simulink model "inverter_fault_rem_sim"  (R2016a)
settings: Solver=ode4  StartTime=0.0  StopTime=Tfinal  FixedStep=Ts  RelTol=1e-3
values from neighbouring files (symbols this model uses):
  Cdc = 200e-6    (= 0.0002)    [inverter_fault_sim.m]
  delta = acos(Ef/Vt)    [inverter_fault_sim.m]
  Ef = 160    [inverter_fault_sim.m]
  Foct = 0    [inverter_fault_sim.m]
  Focw = 1    [inverter_fault_sim.m]
  fout = Nr*p/60    (= 100)    [inverter_fault_sim.m]
  Fsct = 0    [inverter_fault_sim.m]
  Fscw = 0    [inverter_fault_sim.m]
  Ls = 3e-3    (= 0.003)    [inverter_fault_sim.m]    (also in short_circuit.m = 0.00365)
  ma = Vt*sqrt(3)/(Vdcm*0.612)    [inverter_fault_sim.m]
  phase = 0*pi/180    (= 0)    [fault_tolerance_torque.m]    (also in inverter_fault_sim.m = [0 90 0 90])
  Rin = 10    [inverter_fault_sim.m]
  Ripth = 0.15    [inverter_fault_sim.m]
  Rs = 0.277e-6    (= 2.77e-07)    [inverter_fault_sim.m]    (also in short_circuit.m = 0.277)
  Tfault = 0    [inverter_fault_sim.m]
  Ts = 1e-6    (= 1e-06)    [inverter_fault_sim.m]
  Vin = Vdc + Rin*(Pout/Vdc)    (= 688.148148148)    [inverter_fault_sim.m]
  wm = Nm*2*pi/60    (= 62.8318530718)    [fault_tolerance_torque.m]    (also in inverter_fault_sim.m)
  wout = 2*pi*fout    (= 628.318530718)    [inverter_fault_sim.m]
undefined symbols (not defined in the file or in its folder): Lload, Rload
libraries: powerlib x35, powerlib_meascontrol x7, simulink x2
settings Model: Creator=ugurm  LastModifiedBy=mesutto
settings DataIOCC: LimitDataPoints=on  SaveFormat=Array
settings DebuggingCC: UnderspecifiedInitializationDetection=Classic  MergeDetectMultiDrivingBlocksExec=none  SolverPrmCheckMsg=warning  StateNameClashWarn=warning
settings HardwareCC: ProdBitPerPointer=32  ProdLargestAtomicFloat=None  ProdIntDivRoundTo=Undefined  ProdEndianess=Unspecified  ProdWordSize=32  ProdHWDeviceType=32-bit Generic
settings ModelReferenceCC: PropagateSignalLabelsOutOfModel=off
settings ConfigComp: CovModelRefEnable=Off

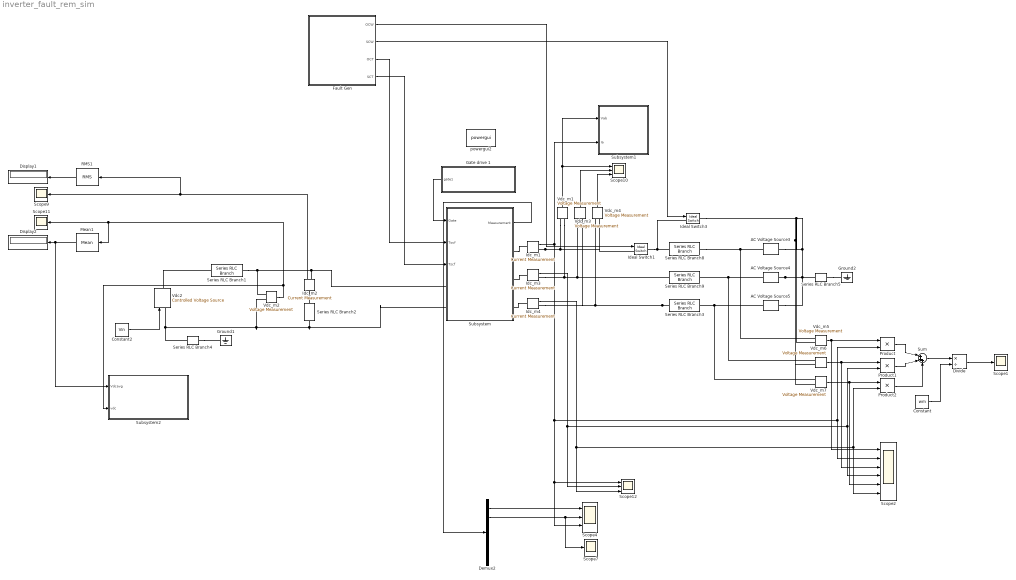
== system inverter_fault_rem_sim ==
  AC Voltage Source3 : powerlib/Electrical Sources/AC Voltage Source  Amplitude=Ef*sqrt(2)  Phase=0  Frequency=fout  SampleTime=0  Measurements=None  BusType=swing  Pref=10e3  Qref=0  Qmin=-inf  Qmax=+inf
  AC Voltage Source4 : powerlib/Electrical Sources/AC Voltage Source  Amplitude=Ef*sqrt(2)  Phase=-120  Frequency=fout  SampleTime=0  Measurements=None  BusType=swing  Pref=10e3  Qref=0  Qmin=-inf  Qmax=+inf
  AC Voltage Source5 : powerlib/Electrical Sources/AC Voltage Source  Amplitude=Ef*sqrt(2)  Phase=-240  Frequency=fout  SampleTime=0  Measurements=None  BusType=swing  Pref=10e3  Qref=0  Qmin=-inf  Qmax=+inf
  Constant : Constant  Value=wm
  Constant2 : Constant  Value=Vin
  Demux2 : Demux  Outputs=12
  Display1 : Display
  Display2 : Display
  Divide : Product  Inputs=*/
  Fault Gen : Subsystem
  Gate drive 1 : Subsystem
  Ground1 : powerlib/Elements/Ground  LConnTagsString=a
  Ground2 : powerlib/Elements/Ground  LConnTagsString=a
  Idc_m{1..4} (4 alike) : powerlib/Measurements/Current Measurement  PhasorSimulation=off  OutputType=Complex  PSBequivalent=0
  Ideal Switch1 : powerlib/Power Electronics/Ideal Switch  Ron=0.001  Lon=0  IC=0  Rs=1e9  Cs=inf  Measurements=off
  Ideal Switch3 : powerlib/Power Electronics/Ideal Switch  Ron=0.001  Lon=0  IC=0  Rs=1e9  Cs=inf  Measurements=off
  Mean1 : powerlib_meascontrol/Measurements/Mean  Freq=fout  Vinit=0  Ts=0
  Product : Product
  Product1 : Product
  Product2 : Product
  RMS1 : powerlib_meascontrol/Measurements/RMS  TrueRMS=on  Freq=fout  RMSInit=0  Ts=0
  Scope{1,7,9,11} (4 alike) : Scope
  Scope10 : Scope  NumInputPorts=3
  Scope12 : Scope  NumInputPorts=3
  Scope2 : Scope  NumInputPorts=6
  Scope4 : Scope  NumInputPorts=3
  Series RLC Branch1 : powerlib/Elements/Series RLC Branch  LConnTagsString=__new0  RConnTagsString=__new0  BranchType=R  Resistance=Rin  Inductance=Lload  SetiL0=off  InitialCurrent=0  Capacitance=1e-6  Setx0=off  InitialVoltage=0  Measurements=None
  Series RLC Branch2 : powerlib/Elements/Series RLC Branch  LConnTagsString=__new0  RConnTagsString=__new0  BranchType=C  Resistance=Rload  Inductance=Lload  SetiL0=off  InitialCurrent=0  Capacitance=Cdc  Setx0=off  InitialVoltage=0  Measurements=None
  Series RLC Branch3 : powerlib/Elements/Series RLC Branch  LConnTagsString=__new0  RConnTagsString=__new0  BranchType=RL  Resistance=Rs  Inductance=Ls  SetiL0=off  InitialCurrent=0  Capacitance=1e-6  Setx0=off  InitialVoltage=0  Measurements=None
  Series RLC Branch4 : powerlib/Elements/Series RLC Branch  LConnTagsString=__new0  RConnTagsString=__new0  BranchType=R  Resistance=1e12  Inductance=Lload  SetiL0=off  InitialCurrent=0  Capacitance=1e-6  Setx0=off  InitialVoltage=0  Measurements=None
  Series RLC Branch5 : powerlib/Elements/Series RLC Branch  LConnTagsString=__new0  RConnTagsString=__new0  BranchType=R  Resistance=1e12  Inductance=Lload  SetiL0=off  InitialCurrent=0  Capacitance=1e-6  Setx0=off  InitialVoltage=0  Measurements=None
  Series RLC Branch8 : powerlib/Elements/Series RLC Branch  LConnTagsString=__new0  RConnTagsString=__new0  BranchType=RL  Resistance=Rs  Inductance=Ls  SetiL0=off  InitialCurrent=0  Capacitance=1e-6  Setx0=off  InitialVoltage=0  Measurements=None
  Series RLC Branch9 : powerlib/Elements/Series RLC Branch  LConnTagsString=__new0  RConnTagsString=__new0  BranchType=RL  Resistance=Rs  Inductance=Ls  SetiL0=off  InitialCurrent=0  Capacitance=1e-6  Setx0=off  InitialVoltage=0  Measurements=None
  Subsystem : Subsystem
  Subsystem1 : Subsystem
  Subsystem2 : Subsystem
  Sum : Sum  Inputs=|+++
  Vdc2 : powerlib/Electrical Sources/Controlled Voltage Source  Initialize=off  Source_Type=DC  Amplitude=200  Phase=0  Frequency=0  Measurements=None
  Vdc_m{1..7} (7 alike) : powerlib/Measurements/Voltage Measurement  PhasorSimulation=off  OutputType=Complex  PSBequivalent=0
  powergui2 : powerlib/powergui  Priority=1  SimulationMode=Discrete  SolverType=Tustin  SampleTime=Ts  frequency=60  SPID=off  DisableSnubberDevices=off  DisableRonSwitches=off  DisableVfSwitches=off  SwTol=0  DisplayEquations=off  Interpol=off  ExternalGateDelay=off  methode=off  Ts=0  FunctionMessages=off  echomessages=off  HookPort=off  EnableUseOfTLC=off  x0status=blocks  frequencyindice=0  Pbase=100e6  ErrMax=1e-4  Iterations=50  UnitsV=kV  UnitsW=MW  buscounter=0  RestoreLinks=warning  ResistiveCurrentMeasurement=off  Frange=[0:2:500]  Ylog=off  Xlog=on  ShowGrid=off  save=off  variable=ZData  structure=Vdc  ZoomFFT=off  StartTime=0.04  cycles=5  DisplayStyle=5  fundamental=50  FreqAxis=off  MaxFrequency=30000  frequencyindicesteady=1  RmsSteady=1  display=off
  wires:
  Gate drive 1/1(gate1) -> Subsystem/1(Gate)
  Vdc_m1/1 -> Subsystem1/1(Vab), Scope10/1
  Idc_m1/1 -> Subsystem1/2(Ia), Product/2, Scope2/2, Scope4/3, Scope12/1
  Constant2/1 -> Vdc2/1
  Idc_m2/1 -> RMS1/1, Scope9/1
  Vdc_m2/1 -> Subsystem2/2(vdc), Mean1/1, Scope11/1
  Idc_m3/1 -> Scope12/2, Product1/2, Scope2/4
  Idc_m4/1 -> Product2/2, Scope2/6, Scope12/3
  RMS1/1 -> Display1/1
  Vdc_m3/1 -> Scope10/2
  Vdc_m4/1 -> Scope10/3
  Mean1/1 -> Subsystem2/1(Vdcavg), Display2/1
  Demux2/1 -> Scope4/1
  Demux2/3 -> Scope7/1, Scope4/2
  Subsystem/1(Measurement) -> Demux2/1
  Fault Gen/4(SCT) -> Subsystem/3(Tscf)
  Fault Gen/3(OCT) -> Subsystem/2(Tocf)
  Fault Gen/2(SCW) -> Ideal Switch3/1
  Fault Gen/1(OCW) -> Ideal Switch1/1
  Vdc_m5/1 -> Scope2/1, Product/1
  Vdc_m6/1 -> Scope2/3, Product1/1
  Vdc_m7/1 -> Scope2/5, Product2/1
  Product1/1 -> Sum/2
  Product2/1 -> Sum/3
  Product/1 -> Sum/1
  Sum/1 -> Divide/1
  Constant/1 -> Divide/2
  Divide/1 -> Scope1/1
  connections:
  Idc_m1/RConn1 -- Ideal Switch1/LConn1 -- Vdc_m4/LConn2 -- Vdc_m1/LConn1
  Series RLC Branch2/RConn1 -- Subsystem/LConn2 -- Vdc_m2/LConn2 -- Series RLC Branch4/LConn1 -- Vdc2/LConn1
  Series RLC Branch1/RConn1 -- Vdc_m2/LConn1 -- Subsystem/LConn1 -- Idc_m2/RConn1
  AC Voltage Source4/LConn1 -- Ideal Switch3/RConn1 -- Vdc_m7/LConn2 -- Vdc_m6/LConn2 -- Vdc_m5/LConn2 -- AC Voltage Source3/LConn1 -- Series RLC Branch5/LConn1 -- AC Voltage Source5/LConn1
  Series RLC Branch3/LConn1 -- Vdc_m4/LConn1 -- Idc_m4/RConn1 -- Vdc_m3/LConn2
  Vdc_m1/LConn2 -- Idc_m3/RConn1 -- Vdc_m3/LConn1 -- Series RLC Branch9/LConn1
  Subsystem/RConn1 -- Idc_m1/LConn1
  Idc_m4/LConn1 -- Subsystem/RConn3
  Series RLC Branch4/RConn1 -- Ground1/LConn1
  AC Voltage Source4/RConn1 -- Vdc_m6/LConn1 -- Series RLC Branch9/RConn1
  Idc_m3/LConn1 -- Subsystem/RConn2
  Idc_m2/LConn1 -- Series RLC Branch2/LConn1
  Vdc2/RConn1 -- Series RLC Branch1/LConn1
  AC Voltage Source5/RConn1 -- Vdc_m7/LConn1 -- Series RLC Branch3/RConn1
  Series RLC Branch5/RConn1 -- Ground2/LConn1
  Series RLC Branch8/RConn1 -- Vdc_m5/LConn1 -- AC Voltage Source3/RConn1
  Ideal Switch1/RConn1 -- Ideal Switch3/LConn1 -- Series RLC Branch8/LConn1

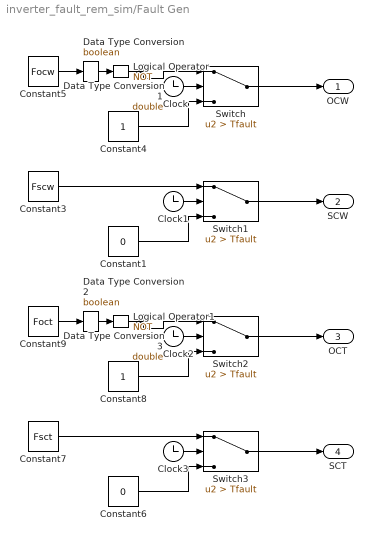
== system inverter_fault_rem_sim/Fault Gen ==
  Clock{,1..3} (4 alike) : Clock
  Constant1 : Constant  Value=0
  Constant3 : Constant  Value=Fscw
  Constant4 : Constant
  Constant5 : Constant  Value=Focw
  Constant6 : Constant  Value=0
  Constant7 : Constant  Value=Fsct
  Constant8 : Constant
  Constant9 : Constant  Value=Foct
  Data Type Conversion : DataTypeConversion  OutDataTypeStr=boolean
  Data Type Conversion1 : DataTypeConversion  OutDataTypeStr=double
  Data Type Conversion2 : DataTypeConversion  OutDataTypeStr=boolean
  Data Type Conversion3 : DataTypeConversion  OutDataTypeStr=double
  Logical Operator : Logic  Operator=NOT  AllPortsSameDT=off  OutDataTypeStr=boolean
  Logical Operator1 : Logic  Operator=NOT  AllPortsSameDT=off  OutDataTypeStr=boolean
  Switch{,1..3} (4 alike) : Switch  Criteria=u2 > Threshold  Threshold=Tfault
  OCW : Outport
  SCW : Outport  Port=2
  OCT : Outport  Port=3
  SCT : Outport  Port=4
  wires:
  Data Type Conversion1/1 -> Switch/1
  Data Type Conversion/1 -> Logical Operator/1
  Logical Operator/1 -> Data Type Conversion1/1
  Constant5/1 -> Data Type Conversion/1
  Constant1/1 -> Switch1/3
  Constant3/1 -> Switch1/1
  Clock1/1 -> Switch1/2
  Switch1/1 -> SCW/1
  Switch/1 -> OCW/1
  Constant4/1 -> Switch/3
  Clock/1 -> Switch/2
  Clock2/1 -> Switch2/2
  Clock3/1 -> Switch3/2
  Constant6/1 -> Switch3/3
  Switch2/1 -> OCT/1
  Data Type Conversion3/1 -> Switch2/1
  Constant9/1 -> Data Type Conversion2/1
  Constant8/1 -> Switch2/3
  Logical Operator1/1 -> Data Type Conversion3/1
  Data Type Conversion2/1 -> Logical Operator1/1
  Constant7/1 -> Switch3/1
  Switch3/1 -> SCT/1

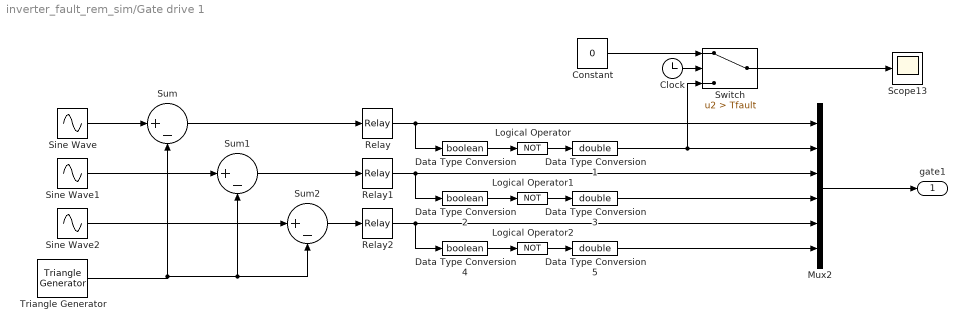
== system inverter_fault_rem_sim/Gate drive 1 ==
  Clock : Clock
  Constant : Constant  Value=0
  Data Type Conversion : DataTypeConversion  OutDataTypeStr=boolean
  Data Type Conversion1 : DataTypeConversion  OutDataTypeStr=double
  Data Type Conversion2 : DataTypeConversion  OutDataTypeStr=boolean
  Data Type Conversion3 : DataTypeConversion  OutDataTypeStr=double
  Data Type Conversion4 : DataTypeConversion  OutDataTypeStr=boolean
  Data Type Conversion5 : DataTypeConversion  OutDataTypeStr=double
  Logical Operator : Logic  Operator=NOT  AllPortsSameDT=off  OutDataTypeStr=boolean
  Logical Operator1 : Logic  Operator=NOT  AllPortsSameDT=off  OutDataTypeStr=boolean
  Logical Operator2 : Logic  Operator=NOT  AllPortsSameDT=off  OutDataTypeStr=boolean
  Mux2 : Mux  Inputs=6
  Relay : Relay
  Relay1 : Relay
  Relay2 : Relay
  Scope13 : Scope
  Sine Wave : Sin  Amplitude=ma  Frequency=wout  Phase=delta  SampleTime=0
  Sine Wave1 : Sin  Amplitude=ma  Frequency=wout  Phase=-2*pi/3+delta  SampleTime=0
  Sine Wave2 : Sin  Amplitude=ma  Frequency=wout  Phase=2*pi/3+delta  SampleTime=0
  Sum : Sum  Inputs=|+-
  Sum1 : Sum  Inputs=|+-
  Sum2 : Sum  Inputs=|+-
  Switch : Switch  Criteria=u2 > Threshold  Threshold=Tfault
  Triangle Generator : powerlib_meascontrol/Pulse & Signal Generators/Triangle Generator  Freq=fsw  Phase=phase(1)  Ts=Ts
  gate1 : Outport
  wires:
  Sine Wave/1 -> Sum/1
  Triangle Generator/1 -> Sum1/2, Sum2/2, Sum/2
  Sine Wave1/1 -> Sum1/1
  Sine Wave2/1 -> Sum2/1
  Sum/1 -> Relay/1
  Sum1/1 -> Relay1/1
  Sum2/1 -> Relay2/1
  Data Type Conversion/1 -> Logical Operator/1
  Relay/1 -> Data Type Conversion/1, Mux2/1
  Logical Operator/1 -> Data Type Conversion1/1
  Data Type Conversion2/1 -> Logical Operator1/1
  Relay1/1 -> Data Type Conversion2/1, Mux2/3
  Logical Operator1/1 -> Data Type Conversion3/1
  Data Type Conversion3/1 -> Mux2/4
  Data Type Conversion4/1 -> Logical Operator2/1
  Relay2/1 -> Data Type Conversion4/1, Mux2/5
  Logical Operator2/1 -> Data Type Conversion5/1
  Data Type Conversion5/1 -> Mux2/6
  Mux2/1 -> gate1/1
  Clock/1 -> Switch/2
  Switch/1 -> Scope13/1
  Constant/1 -> Switch/1
  Data Type Conversion1/1 -> Mux2/2, Switch/3

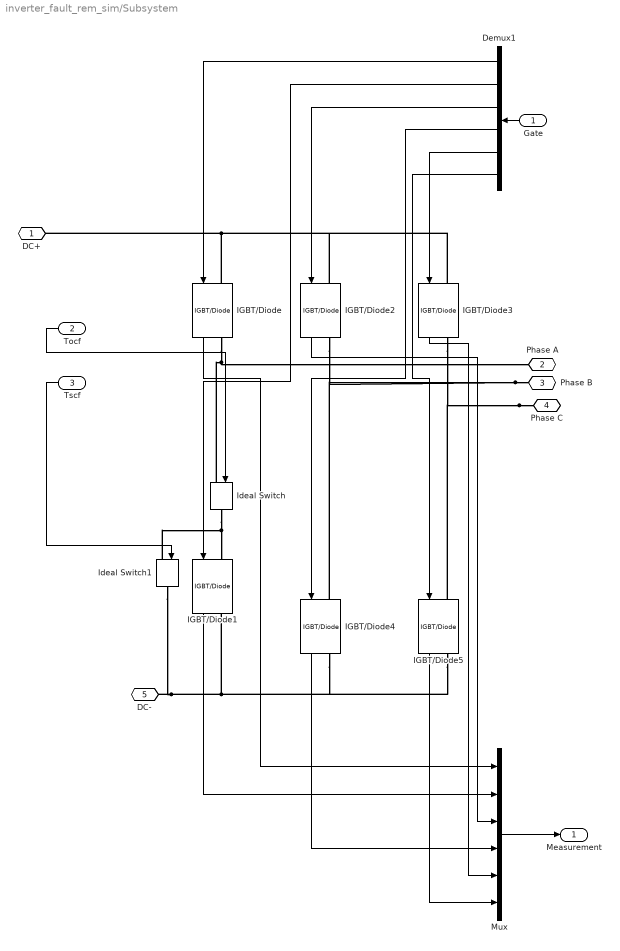
== system inverter_fault_rem_sim/Subsystem ==
  Gate : Inport
  Tocf : Inport  Port=2
  Tscf : Inport  Port=3
  Demux1 : Demux  Outputs=6
  IGBT/Diode{,1..5} (6 alike) : powerlib/Power Electronics/IGBT//Diode  Ron=1e-3  Rs=1e5  Cs=inf  Measurements=on
  Ideal Switch : powerlib/Power Electronics/Ideal Switch  Ron=0.001  Lon=0  IC=0  Rs=inf  Cs=inf  Measurements=off
  Ideal Switch1 : powerlib/Power Electronics/Ideal Switch  Ron=0.001  Lon=0  IC=0  Rs=inf  Cs=inf  Measurements=off
  Mux : Mux  Inputs=6
  DC+ : PMIOPort  Port=1  Side=Left
  Phase A : PMIOPort  Port=2  Side=Right
  Phase B : PMIOPort  Port=3  Side=Right
  Phase C : PMIOPort  Port=4  Side=Right
  DC- : PMIOPort  Port=5  Side=Left
  Measurement : Outport
  wires:
  Gate/1 -> Demux1/1
  Demux1/4 -> IGBT/Diode4/1
  Demux1/2 -> IGBT/Diode1/1
  Demux1/3 -> IGBT/Diode2/1
  Demux1/5 -> IGBT/Diode3/1
  Demux1/6 -> IGBT/Diode5/1
  Demux1/1 -> IGBT/Diode/1
  IGBT/Diode/1 -> Mux/1
  IGBT/Diode1/1 -> Mux/2
  IGBT/Diode2/1 -> Mux/3
  IGBT/Diode4/1 -> Mux/4
  IGBT/Diode3/1 -> Mux/5
  IGBT/Diode5/1 -> Mux/6
  Mux/1 -> Measurement/1
  Tocf/1 -> Ideal Switch/1
  Tscf/1 -> Ideal Switch1/1
  connections:
  Phase C/RConn1 -- IGBT/Diode5/LConn1 -- IGBT/Diode3/RConn1
  IGBT/Diode3/LConn1 -- IGBT/Diode2/LConn1 -- IGBT/Diode/LConn1 -- DC+/RConn1
  IGBT/Diode5/RConn1 -- IGBT/Diode4/RConn1 -- IGBT/Diode1/RConn1 -- Ideal Switch1/RConn1 -- DC-/RConn1
  IGBT/Diode/RConn1 -- Ideal Switch/LConn1 -- Phase A/RConn1
  Phase B/RConn1 -- IGBT/Diode4/LConn1 -- IGBT/Diode2/RConn1
  Ideal Switch/RConn1 -- Ideal Switch1/LConn1 -- IGBT/Diode1/LConn1

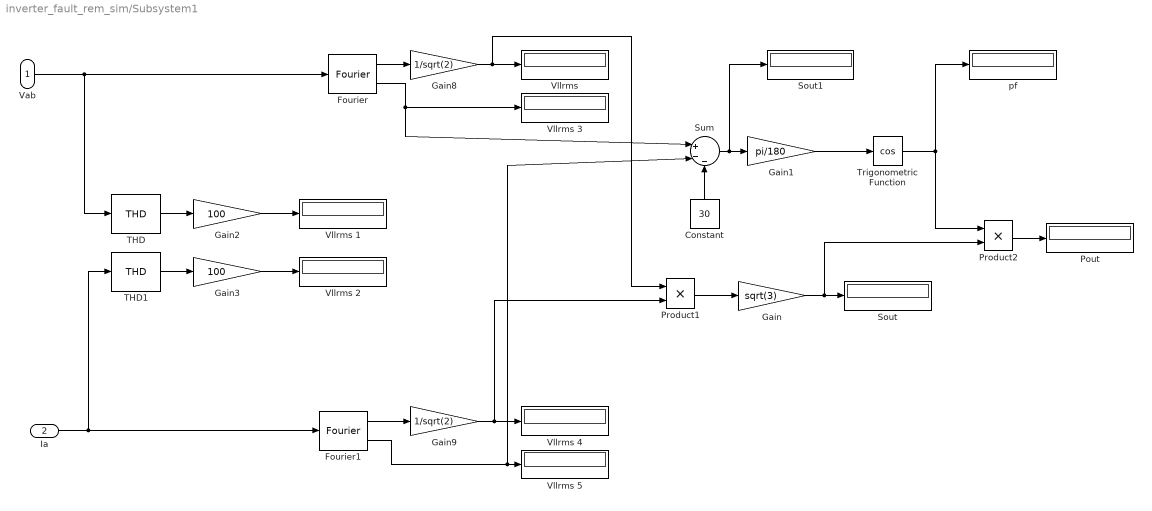
== system inverter_fault_rem_sim/Subsystem1 ==
  Vab : Inport
  Ia : Inport  Port=2
  Constant : Constant  Value=30
  Fourier : powerlib_meascontrol/Measurements/Fourier  Freq=fout  n=1  InInit=[0, 0]  Ts=Ts
  Fourier1 : powerlib_meascontrol/Measurements/Fourier  Freq=fout  n=1  InInit=[0, 0]  Ts=Ts
  Gain : Gain  Gain=sqrt(3)
  Gain1 : Gain  Gain=pi/180
  Gain2 : Gain  Gain=100
  Gain3 : Gain  Gain=100
  Gain8 : Gain  Gain=1/sqrt(2)
  Gain9 : Gain  Gain=1/sqrt(2)
  Pout : Display
  Product1 : Product
  Product2 : Product
  Sout : Display
      settings: Format=short_e
  Sout1 : Display
      settings: Format=short_e
  Sum : Sum  Inputs=|+--
  THD : powerlib_meascontrol/Measurements/THD  Freq=fout  Ts=0
  THD1 : powerlib_meascontrol/Measurements/THD  Freq=fout  Ts=0
  Trigonometric Function : Trigonometry  Operator=cos
  Vllrms {,1..5} (6 alike) : Display
  pf : Display
  wires:
  Gain8/1 -> "Vllrms "/1, Product1/1
  Gain9/1 -> Vllrms 4/1, Product1/2
  Ia/1 -> Fourier1/1, THD1/1
  Fourier1/1 -> Gain9/1
  Vab/1 -> Fourier/1, THD/1
  Fourier/1 -> Gain8/1
  Product1/1 -> Gain/1
  Gain1/1 -> Trigonometric Function/1
  Product2/1 -> Pout/1
  Fourier/2 -> Sum/1, Vllrms 3/1
  THD/1 -> Gain2/1
  THD1/1 -> Gain3/1
  Fourier1/2 -> Sum/2, Vllrms 5/1
  Gain2/1 -> Vllrms 1/1
  Gain3/1 -> Vllrms 2/1
  Gain/1 -> Product2/2, Sout/1
  Sum/1 -> Sout1/1, Gain1/1
  Constant/1 -> Sum/3
  Trigonometric Function/1 -> pf/1, Product2/1

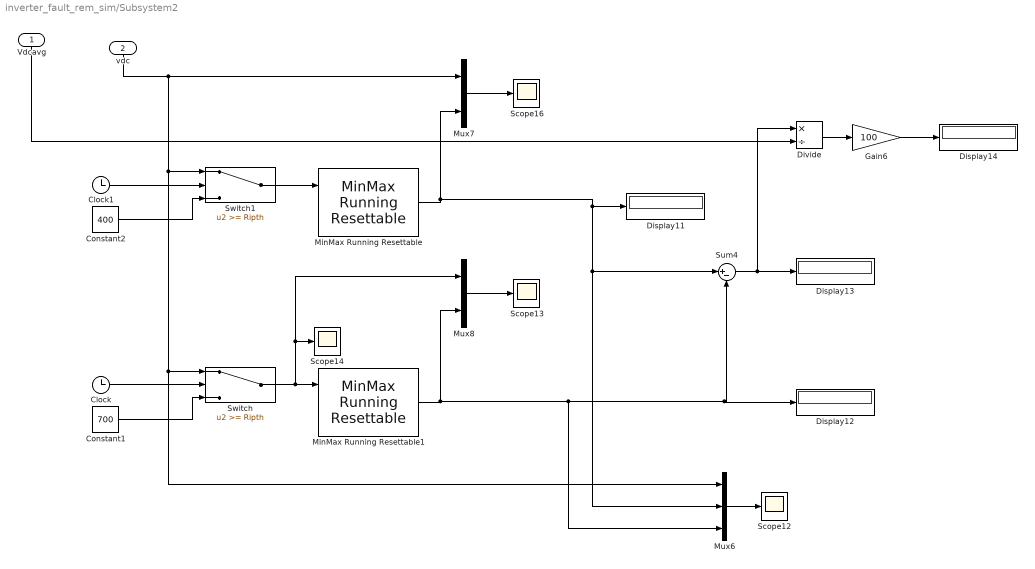
== system inverter_fault_rem_sim/Subsystem2 ==
  Vdcavg : Inport
  vdc : Inport  Port=2
  Clock : Clock
  Clock1 : Clock
  Constant1 : Constant  Value=700  SampleTime=Ts
  Constant2 : Constant  Value=400  SampleTime=Ts
  Display{11..14} (4 alike) : Display
  Divide : Product  Inputs=*/
  Gain6 : Gain  Gain=100
  MinMax Running Resettable : simulink/Math Operations/MinMax Running Resettable  Function=max  vinit=0.0
  MinMax Running Resettable1 : simulink/Math Operations/MinMax Running Resettable  Function=min  vinit=700
  Mux6 : Mux  Inputs=3
  Mux7 : Mux  Inputs=2
  Mux8 : Mux  Inputs=2
  Scope{12..14,16} (4 alike) : Scope
  Sum4 : Sum  Inputs=|+-
  Switch : Switch  Threshold=Ripth
  Switch1 : Switch  Threshold=Ripth
  wires:
  MinMax Running Resettable/1 -> Display11/1, Mux6/2, Sum4/1, Mux7/2
  Clock/1 -> Switch/2
  Mux8/1 -> Scope13/1
  Gain6/1 -> Display14/1
  Constant1/1 -> Switch/3
  MinMax Running Resettable1/1 -> Mux6/3, Display12/1, Sum4/2, Mux8/2
  Mux7/1 -> Scope16/1
  Switch/1 -> Mux8/1, Scope14/1, MinMax Running Resettable1/1
  Sum4/1 -> Divide/1, Display13/1
  Divide/1 -> Gain6/1
  Mux6/1 -> Scope12/1
  Vdcavg/1 -> Divide/2
  vdc/1 -> Mux7/1, Switch1/1, Mux6/1, Switch/1
  Switch1/1 -> MinMax Running Resettable/1
  Clock1/1 -> Switch1/2
  Constant2/1 -> Switch1/3
